simulink model "FusionMODEL_version1"  (R2018a)
settings: Solver=FixedStepAuto  StartTime=0.0  StopTime=SimulationTime  FixedStep=SamplingTime  RelTol=1e-3
undefined symbols (not defined in the file or in its folder): ACTIVATE_CAM, ACTIVATE_RAD, CAM1_detTimeStamp, CAM1_MeasNoise, CAM1_objClassID, CAM1_PX, CAM1_PY, CAM1_VX, CAM1_VY, CAM2_detTimeStamp, CAM2_MeasNoise, CAM2_objClassID, CAM2_PX, CAM2_PY, CAM2_VX, CAM2_VY, CAM3_detTimeStamp, CAM3_MeasNoise, CAM3_objClassID, CAM3_PX, CAM3_PY, CAM3_VX, CAM3_VY, CAM4_detTimeStamp, CAM4_MeasNoise, CAM4_objClassID, CAM4_PX, CAM4_PY, CAM4_VX, CAM4_VY, CAM5_detTimeStamp, CAM5_MeasNoise, CAM5_objClassID, CAM5_PX, CAM5_PY, CAM5_VX, CAM5_VY, CAM6_detTimeStamp, CAM6_MeasNoise, CAM6_objClassID, CAM6_PX, CAM6_PY, CAM6_VX, CAM6_VY, CAM7_detTimeStamp, CAM7_MeasNoise, CAM7_objClassID, CAM7_PX, CAM7_PY, CAM7_VX, CAM7_VY, CAM8_detTimeStamp, CAM8_MeasNoise, CAM8_objClassID, CAM8_PX, CAM8_PY, CAM8_VX, CAM8_VY, CAM_nMeas, CAM_TYPE ... (+151)
libraries: simulink_extras x2
(part 2 of 6)

== system FusionMODEL_version1/OBJECT_TRACKER_SENSOR_FUSION/SPATIAL_ALLIGNMENT/RADAR_MEASUREMENTS_SPATIAL_ALLIGNMENT/SET_MEASUREMENTS ==
  CTSmeasMAT : Inport
  CTSCovMAT : Inport  Port=2
  CTSRefMAT : Inport  Port=3
  validMeasCount : Inport  Port=4
  Add{,1..4} (5 alike) : Sum
  Assignment1 : Assignment  NumberOfDimensions=2  DiagnosticForDimensions=Warning  IndexOptions=Assign all,Starting index (dialog)  Indices=1,1  OutputSizes=1,1
  Assignment2 : Assignment  NumberOfDimensions=3  DiagnosticForDimensions=Warning  IndexOptions=Assign all,Assign all,Starting index (dialog)  Indices=1,1,1  OutputSizes=1,1,1
  Assignment3 : Assignment  NumberOfDimensions=2  DiagnosticForDimensions=Warning  IndexOptions=Assign all,Starting index (dialog)  Indices=1,1  OutputSizes=1,1
  Bus Creator1 : BusCreator  Inputs=5  OutDataTypeStr=Bus: RAD_MEAS_MAT_CTS  NonVirtualBus=on
  Find Nonzero Elements1 : Find  NumberOfInputDimensions=3
  FindNonZeroIndex : MATLAB Function  Commented=on  TreatAsAtomicUnit=on
  Mux1 : Mux  Inputs=6
  Reshape1 : Reshape  OutputDimensionality=Row vector (2-D)
  Selector : Selector  NumberOfDimensions=2  InputPortWidth=3  IndexOptions=Select all,Index vector (dialog)  Indices=1,1  OutputSizes=1,1
  Selector11 : Selector  NumberOfDimensions=2  InputPortWidth=3  IndexOptions=Index vector (dialog),Select all  Indices=1,1  OutputSizes=1,1
  Selector12 : Selector  NumberOfDimensions=2  InputPortWidth=3  IndexOptions=Select all,Index vector (port)  Indices=1,1  OutputSizes=1,1
  Selector14 : Selector  NumberOfDimensions=2  InputPortWidth=3  IndexOptions=Select all,Index vector (port)  Indices=1,1  OutputSizes=1,1
  Selector15 : Selector  NumberOfDimensions=3  InputPortWidth=3  IndexOptions=Select all,Select all,Index vector (port)  Indices=1,1,1  OutputSizes=1,1,1
  Selector2 : Selector  NumberOfDimensions=2  InputPortWidth=3  IndexOptions=Select all,Index vector (dialog)  Indices=5,2  OutputSizes=1,1
  Selector3 : Selector  NumberOfDimensions=2  InputPortWidth=3  IndexOptions=Select all,Index vector (dialog)  Indices=5,3  OutputSizes=1,1
  Selector4 : Selector  NumberOfDimensions=2  InputPortWidth=3  IndexOptions=Select all,Index vector (dialog)  Indices=5,5  OutputSizes=1,1
  Selector5 : Selector  NumberOfDimensions=2  InputPortWidth=3  IndexOptions=Select all,Index vector (dialog)  Indices=6,6  OutputSizes=1,1
  Selector8 : Selector  NumberOfDimensions=2  InputPortWidth=3  IndexOptions=Select all,Index vector (dialog)  Indices=5,4  OutputSizes=1,1
  CTSmeasMATout : Outport
  wires:
  validMeasCount/1 -> Selector2/1, Selector/1, Bus Creator1/4, Selector3/1, Selector8/1, Selector4/1, Selector5/1  "ValidMeasCountMeasCount"
  Add3/1 -> Add4/1, Mux1/5
  Selector3/1 -> Add1/2
  Add2/1 -> Add3/1, Mux1/4
  Add1/1 -> Mux1/3, Add2/1
  Selector4/1 -> Add3/2
  Selector/1 -> Mux1/1, Add/1
  Add/1 -> Add1/1, Mux1/2
  Add4/1 -> Mux1/6
  Selector2/1 -> Add/2
  Selector8/1 -> Add2/2
  Mux1/1 -> Reshape1/1
  Selector5/1 -> Add4/2
  Bus Creator1/1 -> CTSmeasMATout/1
  CTSRefMAT/1 -> [Ref], Selector11/1
  Selector11/1 -> Find Nonzero Elements1/1
  Find Nonzero Elements1/1 -> Selector14/2, Selector12/2, Selector15/2
  CTSmeasMAT/1 -> Assignment1/1, Selector14/1
  Selector14/1 -> Assignment1/2
  Selector15/1 -> Assignment2/2
  Selector12/1 -> Assignment3/2
  CTSCovMAT/1 -> Assignment2/1, Selector15/1
  Assignment3/1 -> Bus Creator1/3  "MeasRef"
  Assignment2/1 -> Bus Creator1/2  "MeasCovariance"
  Assignment1/1 -> Bus Creator1/1  "MeasArray"
  [Ref] -> Assignment3/1, Selector12/1
  Reshape1/1 -> Bus Creator1/5  "ValidCumulativeMeasCount"

== system FusionMODEL_version1/OBJECT_TRACKER_SENSOR_FUSION/SPATIAL_ALLIGNMENT/RADAR_MEASUREMENTS_SPATIAL_ALLIGNMENT/StartingIndexes1 ==
  SnsrCallib : Inport
  CallibrationInfoExtractor : Subsystem
  Subsystem : Subsystem
  StartingIndexes : Outport
  wires:
  CallibrationInfoExtractor/1(R1nMeas) -> Subsystem/1(R1nMeas)
  CallibrationInfoExtractor/2(R2nMeas) -> Subsystem/2(R2nMeas)
  CallibrationInfoExtractor/3(R3nMeas) -> Subsystem/3(R3nMeas)
  CallibrationInfoExtractor/4(R4nMeas) -> Subsystem/4(R4nMeas)
  CallibrationInfoExtractor/5(R5nMeas) -> Subsystem/5(R5nMeas)
  Subsystem/1(StartingIndexes) -> StartingIndexes/1
  SnsrCallib/1 -> CallibrationInfoExtractor/1(SnsrCallib)

== system FusionMODEL_version1/SENSOR_MEASUREMENTS/RADAR_CAMERA_EGO_SENSOR_INTERFACE/CameraSensors/Camera1 ==
  timeIdx : Inport
  nObjCamera : Inport  Port=2
  SensorMeas : Inport  Port=3
  CHECK_IF_DATA_IS_VALID : Subsystem
  GET_DATA : Subsystem
  LOOP_OVER_CAMERAS : ForIterator  ResetStates=reset  IterationSource=external  IterationVariableDataType=int16
  SET_DATA : Subsystem
  Selector : Selector  InputPortWidth=nCameras  IndexOptions=Index vector (dialog)  Indices=1  OutputSizes=1
  C1 : Outport
  wires:
  nObjCamera/1 -> Selector/1
  LOOP_OVER_CAMERAS/1 -> [index]
  GET_DATA/5(OBJ_TYPE) -> SET_DATA/7(OBJ_TYPE)
  [px] -> SET_DATA/2(px)  "px"
  GET_DATA/7(measCaptureTime) -> SET_DATA/9(TIME_STAMP)
  SET_DATA/1(C1) -> C1/1
  [vx] -> SET_DATA/4(vx)  "vx"
  GET_DATA/1(PX) -> CHECK_IF_DATA_IS_VALID/2(px), [px]
  Selector/1 -> LOOP_OVER_CAMERAS/1
  GET_DATA/3(VX) -> CHECK_IF_DATA_IS_VALID/4(vx), [vx]
  timeIdx/1 -> GET_DATA/2(time)
  CHECK_IF_DATA_IS_VALID/1(ID) -> SET_DATA/6(id)
  SensorMeas/1 -> SET_DATA/1(SensorData)
  GET_DATA/6(NOISE_COV) -> SET_DATA/8(NOISE_COV)
  [vy] -> SET_DATA/5(vy)  "vy"
  [py] -> SET_DATA/3(py)  "py"
  GET_DATA/4(VY) -> CHECK_IF_DATA_IS_VALID/5(vy), [vy]
  GET_DATA/2(PY) -> CHECK_IF_DATA_IS_VALID/3(py), [py]
  [index] -> SET_DATA/10(iter), CHECK_IF_DATA_IS_VALID/1(idx), GET_DATA/1(idx)

== system FusionMODEL_version1/SENSOR_MEASUREMENTS/RADAR_CAMERA_EGO_SENSOR_INTERFACE/CameraSensors/Camera2 ==
  timeIdx : Inport
  nObjCamera : Inport  Port=2
  SensorMeas : Inport  Port=3
  ExtractMeasParam1 : Subsystem
  For Iterator : ForIterator  ResetStates=reset  IterationSource=external  IterationVariableDataType=int16
  IsValid2 : Subsystem
  Selector : Selector  InputPortWidth=nCameras  IndexOptions=Starting index (dialog)  Indices=2  OutputSizes=1
  Subsystem1 : Subsystem
  C2 : Outport
  wires:
  ExtractMeasParam1/1(PX) -> IsValid2/2(px), [px]
  ExtractMeasParam1/7(measCaptureTime) -> Subsystem1/9(TIME_STAMP)
  IsValid2/1(ID) -> Subsystem1/6(id)
  [vy] -> Subsystem1/5(vy)  "vy"
  ExtractMeasParam1/6(NOISE_COV) -> Subsystem1/8(NOISE_COV)
  [vx] -> Subsystem1/4(vx)  "vx"
  SensorMeas/1 -> Subsystem1/1(SensorData)
  nObjCamera/1 -> Selector/1
  [py] -> Subsystem1/3(py)  "py"
  For Iterator/1 -> [index]
  [index] -> Subsystem1/10(iter), IsValid2/1(idx), ExtractMeasParam1/1(idx)
  ExtractMeasParam1/4(VY) -> IsValid2/5(vy), [vy]
  [px] -> Subsystem1/2(px)  "px"
  Selector/1 -> For Iterator/1
  ExtractMeasParam1/2(PY) -> IsValid2/3(py), [py]
  Subsystem1/1(C2) -> C2/1
  ExtractMeasParam1/5(OBJ_TYPE) -> Subsystem1/7(OBJ_TYPE)
  timeIdx/1 -> ExtractMeasParam1/2(time)
  ExtractMeasParam1/3(VX) -> IsValid2/4(vx), [vx]

== system FusionMODEL_version1/SENSOR_MEASUREMENTS/RADAR_CAMERA_EGO_SENSOR_INTERFACE/CameraSensors/Camera3 ==
  timeIdx : Inport
  nObjCamera : Inport  Port=2
  SensorMeas : Inport  Port=3
  ExtractMeasParam1 : Subsystem
  For Iterator : ForIterator  ResetStates=reset  IterationSource=external  IterationVariableDataType=int16
  IsValid2 : Subsystem
  Selector : Selector  InputPortWidth=nCameras  IndexOptions=Starting index (dialog)  Indices=3  OutputSizes=1
  Subsystem1 : Subsystem
  C3 : Outport
  wires:
  ExtractMeasParam1/1(PX) -> IsValid2/2(px), [px]
  ExtractMeasParam1/7(measCaptureTime) -> Subsystem1/9(TIME_STAMP)
  IsValid2/1(ID) -> Subsystem1/6(id)
  [vy] -> Subsystem1/5(vy)  "vy"
  ExtractMeasParam1/6(NOISE_COV) -> Subsystem1/8(NOISE_COV)
  [vx] -> Subsystem1/4(vx)  "vx"
  SensorMeas/1 -> Subsystem1/1(SensorData)
  nObjCamera/1 -> Selector/1
  [py] -> Subsystem1/3(py)  "py"
  For Iterator/1 -> [index]
  [index] -> Subsystem1/10(iter), IsValid2/1(idx), ExtractMeasParam1/1(idx)
  ExtractMeasParam1/4(VY) -> IsValid2/5(vy), [vy]
  [px] -> Subsystem1/2(px)  "px"
  Selector/1 -> For Iterator/1
  ExtractMeasParam1/2(PY) -> IsValid2/3(py), [py]
  Subsystem1/1(C3) -> C3/1
  ExtractMeasParam1/5(OBJ_TYPE) -> Subsystem1/7(OBJ_TYPE)
  timeIdx/1 -> ExtractMeasParam1/2(time)
  ExtractMeasParam1/3(VX) -> IsValid2/4(vx), [vx]

== system FusionMODEL_version1/SENSOR_MEASUREMENTS/RADAR_CAMERA_EGO_SENSOR_INTERFACE/CameraSensors/Camera4 ==
  timeIdx : Inport
  nObjCamera : Inport  Port=2
  SensorMeas : Inport  Port=3
  ExtractMeasParam1 : Subsystem
  For Iterator : ForIterator  ResetStates=reset  IterationSource=external  IterationVariableDataType=int16
  IsValid2 : Subsystem
  Selector : Selector  InputPortWidth=nCameras  IndexOptions=Starting index (dialog)  Indices=4  OutputSizes=1
  Subsystem1 : Subsystem
  C4 : Outport
  wires:
  ExtractMeasParam1/1(PX) -> IsValid2/2(px), [px]
  ExtractMeasParam1/7(measCaptureTime) -> Subsystem1/9(TIME_STAMP)
  IsValid2/1(ID) -> Subsystem1/6(id)
  [vy] -> Subsystem1/5(vy)  "vy"
  ExtractMeasParam1/6(NOISE_COV) -> Subsystem1/8(NOISE_COV)
  [vx] -> Subsystem1/4(vx)  "vx"
  SensorMeas/1 -> Subsystem1/1(SensorData)
  nObjCamera/1 -> Selector/1
  [py] -> Subsystem1/3(py)  "py"
  For Iterator/1 -> [index]
  [index] -> Subsystem1/10(iter), IsValid2/1(idx), ExtractMeasParam1/1(idx)
  ExtractMeasParam1/4(VY) -> IsValid2/5(vy), [vy]
  [px] -> Subsystem1/2(px)  "px"
  Selector/1 -> For Iterator/1
  ExtractMeasParam1/2(PY) -> IsValid2/3(py), [py]
  Subsystem1/1(C4) -> C4/1
  ExtractMeasParam1/5(OBJ_TYPE) -> Subsystem1/7(OBJ_TYPE)
  timeIdx/1 -> ExtractMeasParam1/2(time)
  ExtractMeasParam1/3(VX) -> IsValid2/4(vx), [vx]

== system FusionMODEL_version1/SENSOR_MEASUREMENTS/RADAR_CAMERA_EGO_SENSOR_INTERFACE/CameraSensors/Camera5 ==
  timeIdx : Inport
  nObjCamera : Inport  Port=2
  SensorMeas : Inport  Port=3
  ExtractMeasParam1 : Subsystem
  For Iterator : ForIterator  ResetStates=reset  IterationSource=external  IterationVariableDataType=int16
  IsValid2 : Subsystem
  Selector : Selector  InputPortWidth=nCameras  IndexOptions=Starting index (dialog)  Indices=5  OutputSizes=1
  Subsystem1 : Subsystem
  C5 : Outport
  wires:
  ExtractMeasParam1/1(PX) -> IsValid2/2(px), [px]
  ExtractMeasParam1/7(measCaptureTime) -> Subsystem1/9(TIME_STAMP)
  IsValid2/1(ID) -> Subsystem1/6(id)
  [vy] -> Subsystem1/5(vy)  "vy"
  ExtractMeasParam1/6(NOISE_COV) -> Subsystem1/8(NOISE_COV)
  [vx] -> Subsystem1/4(vx)  "vx"
  SensorMeas/1 -> Subsystem1/1(SensorData)
  nObjCamera/1 -> Selector/1
  [py] -> Subsystem1/3(py)  "py"
  For Iterator/1 -> [index]
  [index] -> Subsystem1/10(iter), IsValid2/1(idx), ExtractMeasParam1/1(idx)
  ExtractMeasParam1/4(VY) -> IsValid2/5(vy), [vy]
  [px] -> Subsystem1/2(px)  "px"
  Selector/1 -> For Iterator/1
  ExtractMeasParam1/2(PY) -> IsValid2/3(py), [py]
  Subsystem1/1(C5) -> C5/1
  ExtractMeasParam1/5(OBJ_TYPE) -> Subsystem1/7(OBJ_TYPE)
  timeIdx/1 -> ExtractMeasParam1/2(time)
  ExtractMeasParam1/3(VX) -> IsValid2/4(vx), [vx]

== system FusionMODEL_version1/SENSOR_MEASUREMENTS/RADAR_CAMERA_EGO_SENSOR_INTERFACE/CameraSensors/Camera6 ==
  timeIdx : Inport
  nObjCamera : Inport  Port=2
  SensorMeas : Inport  Port=3
  ExtractMeasParam1 : Subsystem
  For Iterator : ForIterator  ResetStates=reset  IterationSource=external  IterationVariableDataType=int16
  IsValid2 : Subsystem
  Selector : Selector  InputPortWidth=nCameras  IndexOptions=Starting index (dialog)  Indices=6  OutputSizes=1
  Subsystem1 : Subsystem
  C6 : Outport
  wires:
  ExtractMeasParam1/1(PX) -> IsValid2/2(px), [px]
  ExtractMeasParam1/7(measCaptureTime) -> Subsystem1/9(TIME_STAMP)
  IsValid2/1(ID) -> Subsystem1/6(id)
  [vy] -> Subsystem1/5(vy)  "vy"
  ExtractMeasParam1/6(NOISE_COV) -> Subsystem1/8(NOISE_COV)
  [vx] -> Subsystem1/4(vx)  "vx"
  SensorMeas/1 -> Subsystem1/1(SensorData)
  nObjCamera/1 -> Selector/1
  [py] -> Subsystem1/3(py)  "py"
  For Iterator/1 -> [index]
  [index] -> Subsystem1/10(iter), IsValid2/1(idx), ExtractMeasParam1/1(idx)
  ExtractMeasParam1/4(VY) -> IsValid2/5(vy), [vy]
  [px] -> Subsystem1/2(px)  "px"
  Selector/1 -> For Iterator/1
  ExtractMeasParam1/2(PY) -> IsValid2/3(py), [py]
  Subsystem1/1(C6) -> C6/1
  ExtractMeasParam1/5(OBJ_TYPE) -> Subsystem1/7(OBJ_TYPE)
  timeIdx/1 -> ExtractMeasParam1/2(time)
  ExtractMeasParam1/3(VX) -> IsValid2/4(vx), [vx]

== system FusionMODEL_version1/SENSOR_MEASUREMENTS/RADAR_CAMERA_EGO_SENSOR_INTERFACE/CameraSensors/Camera7 ==
  timeIdx : Inport
  nObjCamera : Inport  Port=2
  SensorMeas : Inport  Port=3
  ExtractMeasParam1 : Subsystem
  For Iterator : ForIterator  ResetStates=reset  IterationSource=external  IterationVariableDataType=int16
  IsValid2 : Subsystem
  Selector : Selector  InputPortWidth=nCameras  IndexOptions=Starting index (dialog)  Indices=7  OutputSizes=1
  Subsystem1 : Subsystem
  C7 : Outport
  wires:
  ExtractMeasParam1/1(PX) -> IsValid2/2(px), [px]
  ExtractMeasParam1/7(measCaptureTime) -> Subsystem1/9(TIME_STAMP)
  IsValid2/1(ID) -> Subsystem1/6(id)
  [vy] -> Subsystem1/5(vy)  "vy"
  ExtractMeasParam1/6(NOISE_COV) -> Subsystem1/8(NOISE_COV)
  [vx] -> Subsystem1/4(vx)  "vx"
  SensorMeas/1 -> Subsystem1/1(SensorData)
  nObjCamera/1 -> Selector/1
  [py] -> Subsystem1/3(py)  "py"
  For Iterator/1 -> [index]
  [index] -> Subsystem1/10(iter), IsValid2/1(idx), ExtractMeasParam1/1(idx)
  ExtractMeasParam1/4(VY) -> IsValid2/5(vy), [vy]
  [px] -> Subsystem1/2(px)  "px"
  Selector/1 -> For Iterator/1
  ExtractMeasParam1/2(PY) -> IsValid2/3(py), [py]
  Subsystem1/1(C7) -> C7/1
  ExtractMeasParam1/5(OBJ_TYPE) -> Subsystem1/7(OBJ_TYPE)
  timeIdx/1 -> ExtractMeasParam1/2(time)
  ExtractMeasParam1/3(VX) -> IsValid2/4(vx), [vx]

== system FusionMODEL_version1/SENSOR_MEASUREMENTS/RADAR_CAMERA_EGO_SENSOR_INTERFACE/CameraSensors/Camera8 ==
  timeIdx : Inport
  nObjCamera : Inport  Port=2
  SensorMeas : Inport  Port=3
  ExtractMeasParam1 : Subsystem
  For Iterator : ForIterator  ResetStates=reset  IterationSource=external  IterationVariableDataType=int16
  IsValid2 : Subsystem
  Selector : Selector  InputPortWidth=nCameras  IndexOptions=Starting index (dialog)  Indices=8  OutputSizes=1
  Subsystem1 : Subsystem
  C8 : Outport
  wires:
  ExtractMeasParam1/1(PX) -> IsValid2/2(px), [px]
  ExtractMeasParam1/7(measCaptureTime) -> Subsystem1/9(TIME_STAMP)
  IsValid2/1(ID) -> Subsystem1/6(id)
  [vy] -> Subsystem1/5(vy)  "vy"
  ExtractMeasParam1/6(NOISE_COV) -> Subsystem1/8(NOISE_COV)
  [vx] -> Subsystem1/4(vx)  "vx"
  SensorMeas/1 -> Subsystem1/1(SensorData)
  nObjCamera/1 -> Selector/1
  [py] -> Subsystem1/3(py)  "py"
  For Iterator/1 -> [index]
  [index] -> Subsystem1/10(iter), IsValid2/1(idx), ExtractMeasParam1/1(idx)
  ExtractMeasParam1/4(VY) -> IsValid2/5(vy), [vy]
  [px] -> Subsystem1/2(px)  "px"
  Selector/1 -> For Iterator/1
  ExtractMeasParam1/2(PY) -> IsValid2/3(py), [py]
  Subsystem1/1(C8) -> C8/1
  ExtractMeasParam1/5(OBJ_TYPE) -> Subsystem1/7(OBJ_TYPE)
  timeIdx/1 -> ExtractMeasParam1/2(time)
  ExtractMeasParam1/3(VX) -> IsValid2/4(vx), [vx]

== system FusionMODEL_version1/SENSOR_MEASUREMENTS/RADAR_CAMERA_EGO_SENSOR_INTERFACE/EgoSensors/ExtractMeasParam ==
  timeIdx : Inport
  Constant : Constant  Value=EGO_PX
  Constant1 : Constant  Value=EGO_PY
  Constant2 : Constant  Value=EGO_VX
  Constant3 : Constant  Value=EGO_VY
  Constant4 : Constant  Value=EGO_YAW
  Constant5 : Constant  Value=EGO_YAWRATE
  Constant6 : Constant  Value=EGO_TimeStamp
  Constant7 : Constant  Value=EGO_IgnitionStatus
  EGO_PX : Selector  NumberOfDimensions=2  InputPortWidth=portSize  IndexOptions=Select all,Index vector (port)  Indices=[1 3],1  OutputSizes=1,1
  EGO_PY : Selector  NumberOfDimensions=2  InputPortWidth=portSize  IndexOptions=Select all,Index vector (port)  Indices=[1 3],1  OutputSizes=1,1
  EGO_VX : Selector  NumberOfDimensions=2  InputPortWidth=portSize  IndexOptions=Select all,Index vector (port)  Indices=[1 3],1  OutputSizes=1,1
  EGO_VY : Selector  NumberOfDimensions=2  InputPortWidth=portSize  IndexOptions=Select all,Index vector (port)  Indices=[1 3],1  OutputSizes=1,1
  EGO_YAW : Selector  NumberOfDimensions=2  InputPortWidth=portSize  IndexOptions=Select all,Index vector (port)  Indices=[1 3],1  OutputSizes=1,1
  EGO_YAWRATE : Selector  NumberOfDimensions=2  InputPortWidth=portSize  IndexOptions=Select all,Index vector (port)  Indices=[1 3],1  OutputSizes=1,1
  TIME_STAMP : Selector  NumberOfDimensions=2  InputPortWidth=portSize  IndexOptions=Select all,Index vector (port)  Indices=[1 3],1  OutputSizes=1,1
  TIME_STAMP1 : Selector  NumberOfDimensions=2  InputPortWidth=portSize  IndexOptions=Select all,Index vector (port)  Indices=[1 3],1  OutputSizes=1,1
  EgoTimeStamp : Outport
  EgoPx : Outport  Port=2
  EgoPy : Outport  Port=3
  EgoVx : Outport  Port=4
  EgoVy : Outport  Port=5
  EgoYaw : Outport  Port=6
  EgoYawRate : Outport  Port=7
  EgoIgnitionStatus : Outport  Port=8
  wires:
  Constant3/1 -> EGO_VY/1
  Constant2/1 -> EGO_VX/1
  Constant/1 -> EGO_PX/1
  Constant1/1 -> EGO_PY/1
  EGO_VX/1 -> EgoVx/1
  EGO_PX/1 -> EgoPx/1
  timeIdx/1 -> EGO_PX/2, EGO_PY/2, EGO_VX/2, EGO_VY/2, EGO_YAW/2, EGO_YAWRATE/2, TIME_STAMP1/2, TIME_STAMP/2
  Constant4/1 -> EGO_YAW/1
  EGO_YAW/1 -> EgoYaw/1
  Constant6/1 -> TIME_STAMP/1
  TIME_STAMP/1 -> EgoTimeStamp/1
  EGO_YAWRATE/1 -> EgoYawRate/1
  Constant5/1 -> EGO_YAWRATE/1
  EGO_PY/1 -> EgoPy/1
  EGO_VY/1 -> EgoVy/1
  Constant7/1 -> TIME_STAMP1/1
  TIME_STAMP1/1 -> EgoIgnitionStatus/1

== system FusionMODEL_version1/SENSOR_MEASUREMENTS/RADAR_CAMERA_EGO_SENSOR_INTERFACE/RadarSensors/Radar1 ==
  timeIdx : Inport
  nObjRadar : Inport  Port=2
  SensorMeas : Inport  Port=3
  CHECK_IF_DATA_VALID : Subsystem
  GET_DATA : Subsystem
  LOOP_OVER_RADARS : ForIterator  ResetStates=reset  IterationSource=external  IterationVariableDataType=int16
  SET_DATA : Subsystem
  Selector : Selector  InputPortWidth=nRadars  IndexOptions=Starting index (dialog)  Indices=1  OutputSizes=1
  R1 : Outport
  wires:
  nObjRadar/1 -> Selector/1
  LOOP_OVER_RADARS/1 -> [index]
  [index] -> CHECK_IF_DATA_VALID/1(idx), GET_DATA/1(idx), SET_DATA/10(iter)
  timeIdx/1 -> GET_DATA/2(time)
  GET_DATA/1(PX) -> CHECK_IF_DATA_VALID/2(px), [px]
  GET_DATA/2(PY) -> CHECK_IF_DATA_VALID/3(py), [py]
  GET_DATA/3(VX) -> CHECK_IF_DATA_VALID/4(vx), [vx]
  GET_DATA/4(VY) -> CHECK_IF_DATA_VALID/5(vy), [vy]
  SensorMeas/1 -> SET_DATA/1(SensorData)
  [px] -> SET_DATA/2(px)  "px"
  [py] -> SET_DATA/3(py)  "py"
  [vx] -> SET_DATA/4(vx)  "vx"
  [vy] -> SET_DATA/5(vy)  "vy"
  SET_DATA/1(R1) -> R1/1
  CHECK_IF_DATA_VALID/1(ID) -> SET_DATA/6(id)
  Selector/1 -> LOOP_OVER_RADARS/1
  GET_DATA/5(SNR) -> SET_DATA/7(SNR)
  GET_DATA/6(NOISE_COV) -> SET_DATA/8(NOISE_COV)
  GET_DATA/7(measCaptureTime) -> SET_DATA/9(TIME_STAMP)

== system FusionMODEL_version1/SENSOR_MEASUREMENTS/RADAR_CAMERA_EGO_SENSOR_INTERFACE/RadarSensors/Radar2 ==
  timeIdx : Inport
  nObjRadar : Inport  Port=2
  SensorMeas : Inport  Port=3
  ExtractMeasParam : Subsystem
  For Iterator : ForIterator  ResetStates=reset  IterationSource=external  IterationVariableDataType=int16
  IsValid1 : Subsystem
  Selector : Selector  InputPortWidth=nRadars  IndexOptions=Starting index (dialog)  Indices=2  OutputSizes=1
  Subsystem : Subsystem
  R2 : Outport
  wires:
  [vx] -> Subsystem/4(vx)  "vx"
  Subsystem/1(R2) -> R2/1
  ExtractMeasParam/1(PX) -> IsValid1/2(px), [px]
  IsValid1/1(ID) -> Subsystem/6(id)
  [py] -> Subsystem/3(py)  "py"
  ExtractMeasParam/3(VX) -> IsValid1/4(vx), [vx]
  ExtractMeasParam/6(NOISE_COV) -> Subsystem/8(NOISE_COV)
  ExtractMeasParam/4(VY) -> IsValid1/5(vy), [vy]
  [px] -> Subsystem/2(px)  "px"
  nObjRadar/1 -> Selector/1
  SensorMeas/1 -> Subsystem/1(SensorData)
  timeIdx/1 -> ExtractMeasParam/2(time)
  [index] -> IsValid1/1(idx), ExtractMeasParam/1(idx), Subsystem/10(iter)
  [vy] -> Subsystem/5(vy)  "vy"
  ExtractMeasParam/2(PY) -> IsValid1/3(py), [py]
  For Iterator/1 -> [index]
  ExtractMeasParam/5(SNR) -> Subsystem/7(SNR)
  ExtractMeasParam/7(measCaptureTime) -> Subsystem/9(TIME_STAMP)
  Selector/1 -> For Iterator/1

== system FusionMODEL_version1/SENSOR_MEASUREMENTS/RADAR_CAMERA_EGO_SENSOR_INTERFACE/RadarSensors/Radar3 ==
  timeIdx : Inport
  nObjRadar : Inport  Port=2
  SensorMeas : Inport  Port=3
  ExtractMeasParam : Subsystem
  For Iterator : ForIterator  ResetStates=reset  IterationSource=external  IterationVariableDataType=int16
  IsValid1 : Subsystem
  Selector : Selector  InputPortWidth=nRadars  IndexOptions=Starting index (dialog)  Indices=3  OutputSizes=1
  Subsystem : Subsystem
  R3 : Outport
  wires:
  [vx] -> Subsystem/4(vx)  "vx"
  Subsystem/1(R3) -> R3/1
  ExtractMeasParam/1(PX) -> IsValid1/2(px), [px]
  IsValid1/1(ID) -> Subsystem/6(id)
  [py] -> Subsystem/3(py)  "py"
  ExtractMeasParam/3(VX) -> IsValid1/4(vx), [vx]
  ExtractMeasParam/6(NOISE_COV) -> Subsystem/8(NOISE_COV)
  ExtractMeasParam/4(VY) -> IsValid1/5(vy), [vy]
  [px] -> Subsystem/2(px)  "px"
  nObjRadar/1 -> Selector/1
  SensorMeas/1 -> Subsystem/1(SensorData)
  timeIdx/1 -> ExtractMeasParam/2(time)
  [index] -> IsValid1/1(idx), ExtractMeasParam/1(idx), Subsystem/10(iter)
  [vy] -> Subsystem/5(vy)  "vy"
  ExtractMeasParam/2(PY) -> IsValid1/3(py), [py]
  For Iterator/1 -> [index]
  ExtractMeasParam/5(SNR) -> Subsystem/7(SNR)
  ExtractMeasParam/7(measCaptureTime) -> Subsystem/9(TIME_STAMP)
  Selector/1 -> For Iterator/1

== system FusionMODEL_version1/SENSOR_MEASUREMENTS/RADAR_CAMERA_EGO_SENSOR_INTERFACE/RadarSensors/Radar4 ==
  timeIdx : Inport
  nObjRadar : Inport  Port=2
  SensorMeas : Inport  Port=3
  ExtractMeasParam : Subsystem
  For Iterator : ForIterator  ResetStates=reset  IterationSource=external  IterationVariableDataType=int16
  IsValid1 : Subsystem
  Selector : Selector  InputPortWidth=nRadars  IndexOptions=Starting index (dialog)  Indices=4  OutputSizes=1
  Subsystem : Subsystem
  R4 : Outport
  wires:
  ExtractMeasParam/2(PY) -> IsValid1/3(py), [py]
  [vy] -> Subsystem/5(vy)  "vy"
  [index] -> IsValid1/1(idx), ExtractMeasParam/1(idx), Subsystem/10(iter)
  SensorMeas/1 -> Subsystem/1(SensorData)
  ExtractMeasParam/6(NOISE_COV) -> Subsystem/8(NOISE_COV)
  ExtractMeasParam/4(VY) -> IsValid1/5(vy), [vy]
  ExtractMeasParam/3(VX) -> IsValid1/4(vx), [vx]
  timeIdx/1 -> ExtractMeasParam/2(time)
  IsValid1/1(ID) -> Subsystem/6(id)
  ExtractMeasParam/1(PX) -> IsValid1/2(px), [px]
  [vx] -> Subsystem/4(vx)  "vx"
  Selector/1 -> For Iterator/1
  nObjRadar/1 -> Selector/1
  Subsystem/1(R4) -> R4/1
  ExtractMeasParam/7(measCaptureTime) -> Subsystem/9(TIME_STAMP)
  [px] -> Subsystem/2(px)  "px"
  ExtractMeasParam/5(SNR) -> Subsystem/7(SNR)
  [py] -> Subsystem/3(py)  "py"
  For Iterator/1 -> [index]

== system FusionMODEL_version1/SENSOR_MEASUREMENTS/RADAR_CAMERA_EGO_SENSOR_INTERFACE/RadarSensors/Radar5 ==
  timeIdx : Inport
  nObjRadar : Inport  Port=2
  SensorMeas : Inport  Port=3
  ExtractMeasParam : Subsystem
  For Iterator : ForIterator  ResetStates=reset  IterationSource=external  IterationVariableDataType=int16
  IsValid1 : Subsystem
  Selector : Selector  InputPortWidth=nRadars  IndexOptions=Starting index (dialog)  Indices=5  OutputSizes=1
  Subsystem : Subsystem
  R5 : Outport
  wires:
  ExtractMeasParam/2(PY) -> IsValid1/3(py), [py]
  [vy] -> Subsystem/5(vy)  "vy"
  [index] -> IsValid1/1(idx), ExtractMeasParam/1(idx), Subsystem/10(iter)
  SensorMeas/1 -> Subsystem/1(SensorData)
  ExtractMeasParam/6(NOISE_COV) -> Subsystem/8(NOISE_COV)
  ExtractMeasParam/4(VY) -> IsValid1/5(vy), [vy]
  ExtractMeasParam/3(VX) -> IsValid1/4(vx), [vx]
  timeIdx/1 -> ExtractMeasParam/2(time)
  IsValid1/1(ID) -> Subsystem/6(id)
  ExtractMeasParam/1(PX) -> IsValid1/2(px), [px]
  [vx] -> Subsystem/4(vx)  "vx"
  Selector/1 -> For Iterator/1
  nObjRadar/1 -> Selector/1
  Subsystem/1(R5) -> R5/1
  ExtractMeasParam/7(measCaptureTime) -> Subsystem/9(TIME_STAMP)
  [px] -> Subsystem/2(px)  "px"
  ExtractMeasParam/5(SNR) -> Subsystem/7(SNR)
  [py] -> Subsystem/3(py)  "py"
  For Iterator/1 -> [index]

== system FusionMODEL_version1/SENSOR_MEASUREMENTS/RADAR_CAMERA_EGO_SENSOR_INTERFACE/RadarSensors/Radar6 ==
  timeIdx : Inport
  nObjRadar : Inport  Port=2
  SensorMeas : Inport  Port=3
  ExtractMeasParam : Subsystem
  For Iterator : ForIterator  ResetStates=reset  IterationSource=external  IterationVariableDataType=int16
  IsValid1 : Subsystem
  Selector : Selector  InputPortWidth=nRadars  IndexOptions=Starting index (dialog)  Indices=6  OutputSizes=1
  Subsystem : Subsystem
  R6 : Outport
  wires:
  ExtractMeasParam/2(PY) -> IsValid1/3(py), [py]
  [vy] -> Subsystem/5(vy)  "vy"
  [index] -> IsValid1/1(idx), ExtractMeasParam/1(idx), Subsystem/10(iter)
  SensorMeas/1 -> Subsystem/1(SensorData)
  ExtractMeasParam/6(NOISE_COV) -> Subsystem/8(NOISE_COV)
  ExtractMeasParam/4(VY) -> IsValid1/5(vy), [vy]
  ExtractMeasParam/3(VX) -> IsValid1/4(vx), [vx]
  timeIdx/1 -> ExtractMeasParam/2(time)
  IsValid1/1(ID) -> Subsystem/6(id)
  ExtractMeasParam/1(PX) -> IsValid1/2(px), [px]
  [vx] -> Subsystem/4(vx)  "vx"
  Selector/1 -> For Iterator/1
  nObjRadar/1 -> Selector/1
  Subsystem/1(R6) -> R6/1
  ExtractMeasParam/7(measCaptureTime) -> Subsystem/9(TIME_STAMP)
  [px] -> Subsystem/2(px)  "px"
  ExtractMeasParam/5(SNR) -> Subsystem/7(SNR)
  [py] -> Subsystem/3(py)  "py"
  For Iterator/1 -> [index]

== system FusionMODEL_version1/SENSOR_MEASUREMENTS/RADAR_CAMERA_EGO_SENSOR_INTERFACE/RoadSensors/Camera1 ==
  timeIdx : Inport
  nLines : Inport  Port=2
  CameraLineCoeff : Inport  Port=3
  CHECK_IF_DATA_IS_VALID : Subsystem
  GET_DATA : Subsystem
  LOOP_OVER_CAMERAS : ForIterator  ResetStates=reset  IterationSource=external  IterationVariableDataType=int16
  SET_DATA : Subsystem
  Selector : Selector  InputPortWidth=nCameras  IndexOptions=Index vector (dialog)  Indices=1  OutputSizes=1
  C1 : Outport
  wires:
  nLines/1 -> Selector/1
  LOOP_OVER_CAMERAS/1 -> [index]
  GET_DATA/5(lateralOffset) -> SET_DATA/7(lateralOffset)
  [curv] -> SET_DATA/2(curv)
  GET_DATA/9(measCaptureTime) -> SET_DATA/11(TIME_STAMP)
  SET_DATA/1(C1) -> C1/1
  [curvLen] -> SET_DATA/4(curvLen)
  GET_DATA/1(curvature) -> CHECK_IF_DATA_IS_VALID/2(curvature), [curv]
  Selector/1 -> LOOP_OVER_CAMERAS/1
  GET_DATA/3(curvLength) -> CHECK_IF_DATA_IS_VALID/4(curvLength), [curvLen]
  timeIdx/1 -> GET_DATA/2(time)
  CHECK_IF_DATA_IS_VALID/1(validID) -> SET_DATA/6(ValidID)
  CameraLineCoeff/1 -> SET_DATA/1(CameraLineCoeff)
  GET_DATA/6(xmin) -> SET_DATA/8(xmin)
  [alpha] -> SET_DATA/5(alpha)
  [curvRate] -> SET_DATA/3(curvRate)
  GET_DATA/4(headingAngle) -> CHECK_IF_DATA_IS_VALID/5(HeadingAngle), [alpha]
  GET_DATA/2(curvRate) -> CHECK_IF_DATA_IS_VALID/3(curvatureRate), [curvRate]
  [index] -> CHECK_IF_DATA_IS_VALID/1(LineID), SET_DATA/12(iter), GET_DATA/1(idx)
  GET_DATA/7(xmax) -> SET_DATA/9(xmax)
  GET_DATA/8(lineMarkWidth) -> SET_DATA/10(lineWidth)

== system FusionMODEL_version1/SENSOR_MEASUREMENTS/RADAR_CAMERA_EGO_SENSOR_INTERFACE/RoadSensors/Camera2 ==
  timeIdx : Inport
  nLines : Inport  Port=2
  CameraLineCoeff : Inport  Port=3
  ExtractMeasParam1 : Subsystem
  For Iterator : ForIterator  ResetStates=reset  IterationSource=external  IterationVariableDataType=int16
  IsValid2 : Subsystem
  Selector : Selector  InputPortWidth=nCameras  IndexOptions=Index vector (dialog)  Indices=2  OutputSizes=1
  Subsystem1 : Subsystem
  C1 : Outport
  wires:
  ExtractMeasParam1/7(xmax) -> Subsystem1/9(xmax)
  ExtractMeasParam1/8(lineMarkWidth) -> Subsystem1/10(lineWidth)
  [index] -> IsValid2/1(LineID), Subsystem1/12(iter), ExtractMeasParam1/1(idx)
  timeIdx/1 -> ExtractMeasParam1/2(time)
  ExtractMeasParam1/2(curvRate) -> IsValid2/3(curvatureRate), [curvRate]
  [curvRate] -> Subsystem1/3(curvRate)
  [curv] -> Subsystem1/2(curv)
  ExtractMeasParam1/3(curvLength) -> IsValid2/4(curvLength), [curvLen]
  ExtractMeasParam1/1(curvature) -> IsValid2/2(curvature), [curv]
  Subsystem1/1(C1) -> C1/1
  [curvLen] -> Subsystem1/4(curvLen)
  For Iterator/1 -> [index]
  ExtractMeasParam1/4(headingAngle) -> IsValid2/5(HeadingAngle), [alpha]
  ExtractMeasParam1/5(lateralOffset) -> Subsystem1/7(lateralOffset)
  Selector/1 -> For Iterator/1
  IsValid2/1(validID) -> Subsystem1/6(ValidID)
  ExtractMeasParam1/6(xmin) -> Subsystem1/8(xmin)
  CameraLineCoeff/1 -> Subsystem1/1(CameraLineCoeff)
  nLines/1 -> Selector/1
  ExtractMeasParam1/9(measCaptureTime) -> Subsystem1/11(TIME_STAMP)
  [alpha] -> Subsystem1/5(alpha)

== system FusionMODEL_version1/SENSOR_MEASUREMENTS/RADAR_CAMERA_EGO_SENSOR_INTERFACE/RoadSensors/Camera3 ==
  timeIdx : Inport
  nLines : Inport  Port=2
  CameraLineCoeff : Inport  Port=3
  ExtractMeasParam1 : Subsystem
  For Iterator : ForIterator  ResetStates=reset  IterationSource=external  IterationVariableDataType=int16
  IsValid2 : Subsystem
  Selector : Selector  InputPortWidth=nCameras  IndexOptions=Index vector (dialog)  Indices=3  OutputSizes=1
  Subsystem1 : Subsystem
  C1 : Outport
  wires:
  ExtractMeasParam1/7(xmax) -> Subsystem1/9(xmax)
  ExtractMeasParam1/8(lineMarkWidth) -> Subsystem1/10(lineWidth)
  [index] -> IsValid2/1(LineID), Subsystem1/12(iter), ExtractMeasParam1/1(idx)
  timeIdx/1 -> ExtractMeasParam1/2(time)
  ExtractMeasParam1/2(curvRate) -> IsValid2/3(curvatureRate), [curvRate]
  [curvRate] -> Subsystem1/3(curvRate)
  [curv] -> Subsystem1/2(curv)
  ExtractMeasParam1/3(curvLength) -> IsValid2/4(curvLength), [curvLen]
  ExtractMeasParam1/1(curvature) -> IsValid2/2(curvature), [curv]
  Subsystem1/1(C1) -> C1/1
  [curvLen] -> Subsystem1/4(curvLen)
  For Iterator/1 -> [index]
  ExtractMeasParam1/4(headingAngle) -> IsValid2/5(HeadingAngle), [alpha]
  ExtractMeasParam1/5(lateralOffset) -> Subsystem1/7(lateralOffset)
  Selector/1 -> For Iterator/1
  IsValid2/1(validID) -> Subsystem1/6(ValidID)
  ExtractMeasParam1/6(xmin) -> Subsystem1/8(xmin)
  CameraLineCoeff/1 -> Subsystem1/1(CameraLineCoeff)
  nLines/1 -> Selector/1
  ExtractMeasParam1/9(measCaptureTime) -> Subsystem1/11(TIME_STAMP)
  [alpha] -> Subsystem1/5(alpha)

== system FusionMODEL_version1/SENSOR_MEASUREMENTS/RADAR_CAMERA_EGO_SENSOR_INTERFACE/RoadSensors/Camera4 ==
  timeIdx : Inport
  nLines : Inport  Port=2
  CameraLineCoeff : Inport  Port=3
  ExtractMeasParam1 : Subsystem
  For Iterator : ForIterator  ResetStates=reset  IterationSource=external  IterationVariableDataType=int16
  IsValid2 : Subsystem
  Selector : Selector  InputPortWidth=nCameras  IndexOptions=Index vector (dialog)  Indices=4  OutputSizes=1
  Subsystem1 : Subsystem
  C1 : Outport
  wires:
  ExtractMeasParam1/7(xmax) -> Subsystem1/9(xmax)
  ExtractMeasParam1/8(lineMarkWidth) -> Subsystem1/10(lineWidth)
  [index] -> IsValid2/1(LineID), Subsystem1/12(iter), ExtractMeasParam1/1(idx)
  timeIdx/1 -> ExtractMeasParam1/2(time)
  ExtractMeasParam1/2(curvRate) -> IsValid2/3(curvatureRate), [curvRate]
  [curvRate] -> Subsystem1/3(curvRate)
  [curv] -> Subsystem1/2(curv)
  ExtractMeasParam1/3(curvLength) -> IsValid2/4(curvLength), [curvLen]
  ExtractMeasParam1/1(curvature) -> IsValid2/2(curvature), [curv]
  Subsystem1/1(C1) -> C1/1
  [curvLen] -> Subsystem1/4(curvLen)
  For Iterator/1 -> [index]
  ExtractMeasParam1/4(headingAngle) -> IsValid2/5(HeadingAngle), [alpha]
  ExtractMeasParam1/5(lateralOffset) -> Subsystem1/7(lateralOffset)
  Selector/1 -> For Iterator/1
  IsValid2/1(validID) -> Subsystem1/6(ValidID)
  ExtractMeasParam1/6(xmin) -> Subsystem1/8(xmin)
  CameraLineCoeff/1 -> Subsystem1/1(CameraLineCoeff)
  nLines/1 -> Selector/1
  ExtractMeasParam1/9(measCaptureTime) -> Subsystem1/11(TIME_STAMP)
  [alpha] -> Subsystem1/5(alpha)

== system FusionMODEL_version1/SENSOR_MEASUREMENTS/RADAR_CAMERA_EGO_SENSOR_INTERFACE/RoadSensors/Camera5 ==
  timeIdx : Inport
  nLines : Inport  Port=2
  CameraLineCoeff : Inport  Port=3
  ExtractMeasParam1 : Subsystem
  For Iterator : ForIterator  ResetStates=reset  IterationSource=external  IterationVariableDataType=int16
  IsValid2 : Subsystem
  Selector : Selector  InputPortWidth=nCameras  IndexOptions=Index vector (dialog)  Indices=5  OutputSizes=1
  Subsystem1 : Subsystem
  C1 : Outport
  wires:
  ExtractMeasParam1/7(xmax) -> Subsystem1/9(xmax)
  ExtractMeasParam1/8(lineMarkWidth) -> Subsystem1/10(lineWidth)
  [index] -> IsValid2/1(LineID), Subsystem1/12(iter), ExtractMeasParam1/1(idx)
  timeIdx/1 -> ExtractMeasParam1/2(time)
  ExtractMeasParam1/2(curvRate) -> IsValid2/3(curvatureRate), [curvRate]
  [curvRate] -> Subsystem1/3(curvRate)
  [curv] -> Subsystem1/2(curv)
  ExtractMeasParam1/3(curvLength) -> IsValid2/4(curvLength), [curvLen]
  ExtractMeasParam1/1(curvature) -> IsValid2/2(curvature), [curv]
  Subsystem1/1(C1) -> C1/1
  [curvLen] -> Subsystem1/4(curvLen)
  For Iterator/1 -> [index]
  ExtractMeasParam1/4(headingAngle) -> IsValid2/5(HeadingAngle), [alpha]
  ExtractMeasParam1/5(lateralOffset) -> Subsystem1/7(lateralOffset)
  Selector/1 -> For Iterator/1
  IsValid2/1(validID) -> Subsystem1/6(ValidID)
  ExtractMeasParam1/6(xmin) -> Subsystem1/8(xmin)
  CameraLineCoeff/1 -> Subsystem1/1(CameraLineCoeff)
  nLines/1 -> Selector/1
  ExtractMeasParam1/9(measCaptureTime) -> Subsystem1/11(TIME_STAMP)
  [alpha] -> Subsystem1/5(alpha)

== system FusionMODEL_version1/SENSOR_MEASUREMENTS/RADAR_CAMERA_EGO_SENSOR_INTERFACE/RoadSensors/Camera6 ==
  timeIdx : Inport
  nLines : Inport  Port=2
  CameraLineCoeff : Inport  Port=3
  ExtractMeasParam1 : Subsystem
  For Iterator : ForIterator  ResetStates=reset  IterationSource=external  IterationVariableDataType=int16
  IsValid2 : Subsystem
  Selector : Selector  InputPortWidth=nCameras  IndexOptions=Index vector (dialog)  Indices=6  OutputSizes=1
  Subsystem1 : Subsystem
  C1 : Outport
  wires:
  ExtractMeasParam1/7(xmax) -> Subsystem1/9(xmax)
  ExtractMeasParam1/8(lineMarkWidth) -> Subsystem1/10(lineWidth)
  [index] -> IsValid2/1(LineID), Subsystem1/12(iter), ExtractMeasParam1/1(idx)
  timeIdx/1 -> ExtractMeasParam1/2(time)
  ExtractMeasParam1/2(curvRate) -> IsValid2/3(curvatureRate), [curvRate]
  [curvRate] -> Subsystem1/3(curvRate)
  [curv] -> Subsystem1/2(curv)
  ExtractMeasParam1/3(curvLength) -> IsValid2/4(curvLength), [curvLen]
  ExtractMeasParam1/1(curvature) -> IsValid2/2(curvature), [curv]
  Subsystem1/1(C1) -> C1/1
  [curvLen] -> Subsystem1/4(curvLen)
  For Iterator/1 -> [index]
  ExtractMeasParam1/4(headingAngle) -> IsValid2/5(HeadingAngle), [alpha]
  ExtractMeasParam1/5(lateralOffset) -> Subsystem1/7(lateralOffset)
  Selector/1 -> For Iterator/1
  IsValid2/1(validID) -> Subsystem1/6(ValidID)
  ExtractMeasParam1/6(xmin) -> Subsystem1/8(xmin)
  CameraLineCoeff/1 -> Subsystem1/1(CameraLineCoeff)
  nLines/1 -> Selector/1
  ExtractMeasParam1/9(measCaptureTime) -> Subsystem1/11(TIME_STAMP)
  [alpha] -> Subsystem1/5(alpha)

== system FusionMODEL_version1/SENSOR_MEASUREMENTS/RADAR_CAMERA_EGO_SENSOR_INTERFACE/RoadSensors/Camera7 ==
  timeIdx : Inport
  nLines : Inport  Port=2
  CameraLineCoeff : Inport  Port=3
  ExtractMeasParam1 : Subsystem
  For Iterator : ForIterator  ResetStates=reset  IterationSource=external  IterationVariableDataType=int16
  IsValid2 : Subsystem
  Selector : Selector  InputPortWidth=nCameras  IndexOptions=Index vector (dialog)  Indices=7  OutputSizes=1
  Subsystem1 : Subsystem
  C1 : Outport
  wires:
  ExtractMeasParam1/7(xmax) -> Subsystem1/9(xmax)
  ExtractMeasParam1/8(lineMarkWidth) -> Subsystem1/10(lineWidth)
  [index] -> IsValid2/1(LineID), Subsystem1/12(iter), ExtractMeasParam1/1(idx)
  timeIdx/1 -> ExtractMeasParam1/2(time)
  ExtractMeasParam1/2(curvRate) -> IsValid2/3(curvatureRate), [curvRate]
  [curvRate] -> Subsystem1/3(curvRate)
  [curv] -> Subsystem1/2(curv)
  ExtractMeasParam1/3(curvLength) -> IsValid2/4(curvLength), [curvLen]
  ExtractMeasParam1/1(curvature) -> IsValid2/2(curvature), [curv]
  Subsystem1/1(C1) -> C1/1
  [curvLen] -> Subsystem1/4(curvLen)
  For Iterator/1 -> [index]
  ExtractMeasParam1/4(headingAngle) -> IsValid2/5(HeadingAngle), [alpha]
  ExtractMeasParam1/5(lateralOffset) -> Subsystem1/7(lateralOffset)
  Selector/1 -> For Iterator/1
  IsValid2/1(validID) -> Subsystem1/6(ValidID)
  ExtractMeasParam1/6(xmin) -> Subsystem1/8(xmin)
  CameraLineCoeff/1 -> Subsystem1/1(CameraLineCoeff)
  nLines/1 -> Selector/1
  ExtractMeasParam1/9(measCaptureTime) -> Subsystem1/11(TIME_STAMP)
  [alpha] -> Subsystem1/5(alpha)

== system FusionMODEL_version1/SENSOR_MEASUREMENTS/RADAR_CAMERA_EGO_SENSOR_INTERFACE/RoadSensors/Camera8 ==
  timeIdx : Inport
  nLines : Inport  Port=2
  CameraLineCoeff : Inport  Port=3
  ExtractMeasParam1 : Subsystem
  For Iterator : ForIterator  ResetStates=reset  IterationSource=external  IterationVariableDataType=int16
  IsValid2 : Subsystem
  Selector : Selector  InputPortWidth=nCameras  IndexOptions=Index vector (dialog)  Indices=8  OutputSizes=1
  Subsystem1 : Subsystem
  C1 : Outport
  wires:
  ExtractMeasParam1/7(xmax) -> Subsystem1/9(xmax)
  ExtractMeasParam1/8(lineMarkWidth) -> Subsystem1/10(lineWidth)
  [index] -> IsValid2/1(LineID), Subsystem1/12(iter), ExtractMeasParam1/1(idx)
  timeIdx/1 -> ExtractMeasParam1/2(time)
  ExtractMeasParam1/2(curvRate) -> IsValid2/3(curvatureRate), [curvRate]
  [curvRate] -> Subsystem1/3(curvRate)
  [curv] -> Subsystem1/2(curv)
  ExtractMeasParam1/3(curvLength) -> IsValid2/4(curvLength), [curvLen]
  ExtractMeasParam1/1(curvature) -> IsValid2/2(curvature), [curv]
  Subsystem1/1(C1) -> C1/1
  [curvLen] -> Subsystem1/4(curvLen)
  For Iterator/1 -> [index]
  ExtractMeasParam1/4(headingAngle) -> IsValid2/5(HeadingAngle), [alpha]
  ExtractMeasParam1/5(lateralOffset) -> Subsystem1/7(lateralOffset)
  Selector/1 -> For Iterator/1
  IsValid2/1(validID) -> Subsystem1/6(ValidID)
  ExtractMeasParam1/6(xmin) -> Subsystem1/8(xmin)
  CameraLineCoeff/1 -> Subsystem1/1(CameraLineCoeff)
  nLines/1 -> Selector/1
  ExtractMeasParam1/9(measCaptureTime) -> Subsystem1/11(TIME_STAMP)
  [alpha] -> Subsystem1/5(alpha)

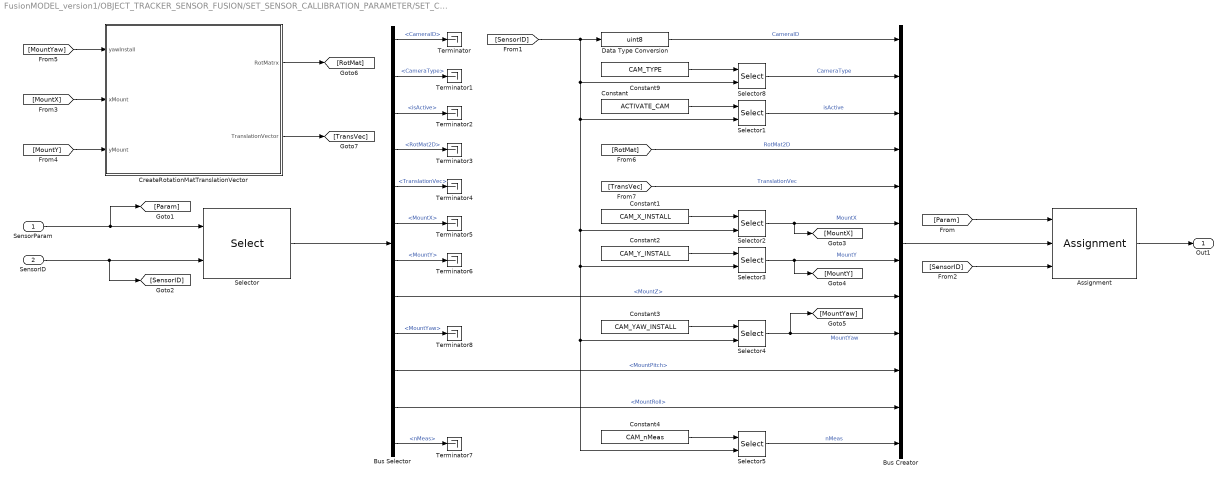
== system FusionMODEL_version1/OBJECT_TRACKER_SENSOR_FUSION/SET_SENSOR_CALLIBRATION_PARAMETER/SET_CAMERA_SENSOR_PARAM/SET_CAMERA_EXTRINSIC_PARAM/SET_CAMERA_EXTRINSIC_PARAM ==
  SensorParam : Inport
  SensorID : Inport  Port=2
  Assignment : Assignment  DiagnosticForDimensions=Warning  IndexOptions=Index vector (port)  Indices=1  OutputSizes=1
  Bus Creator : BusCreator  Inputs=12  OutDataTypeStr=Bus: CameraExtrinsicParam  NonVirtualBus=on
  Bus Selector : BusSelector  OutputSignals=CameraID,CameraType,isActive,RotMat2D,TranslationVec,MountX,MountY,MountZ,MountYaw,MountPitch,MountRoll,nMeas
  Constant : Constant  Value=ACTIVATE_CAM
  Constant1 : Constant  Value=CAM_X_INSTALL
  Constant2 : Constant  Value=CAM_Y_INSTALL
  Constant3 : Constant  Value=CAM_YAW_INSTALL
  Constant4 : Constant  Value=CAM_nMeas
  Constant9 : Constant  Value=CAM_TYPE
  CreateRotationMatTranslationVector : Subsystem
  Data Type Conversion : DataTypeConversion  OutDataTypeStr=uint8
  Selector{,1..5,8} (7 alike) : Selector  InputPortWidth=nCameras  IndexOptions=Index vector (port)  Indices=[1 3]  OutputSizes=1
  Terminator{,1..8} (9 alike) : Terminator
  Out1 : Outport
  wires:
  Assignment/1 -> Out1/1
  Constant/1 -> Selector1/1
  SensorParam/1 -> [Param], Selector/1
  Constant2/1 -> Selector3/1
  [SensorID] -> Selector5/2, Selector4/2, Selector3/2, Selector2/2, Selector1/2, Selector8/2, Data Type Conversion/1
  Constant3/1 -> Selector4/1
  Constant1/1 -> Selector2/1
  Selector/1 -> Bus Selector/1
  Bus Creator/1 -> Assignment/2
  Bus Selector/1 -> Terminator/1  "<CameraID>"
  SensorID/1 -> [SensorID], Selector/2
  [Param] -> Assignment/1
  [SensorID] -> Assignment/3
  Selector2/1 -> [MountX], Bus Creator/6  "MountX"
  Selector3/1 -> [MountY], Bus Creator/7  "MountY"
  [MountX] -> CreateRotationMatTranslationVector/2(xMount)
  [MountY] -> CreateRotationMatTranslationVector/3(yMount)
  Selector4/1 -> [MountYaw], Bus Creator/9  "MountYaw"
  [MountYaw] -> CreateRotationMatTranslationVector/1(yawInstall)
  CreateRotationMatTranslationVector/1(RotMatrx) -> [RotMat]
  CreateRotationMatTranslationVector/2(TranslationVector) -> [TransVec]
  Data Type Conversion/1 -> Bus Creator/1  "CameraID"
  Selector8/1 -> Bus Creator/2  "CameraType"
  Constant9/1 -> Selector8/1
  Selector1/1 -> Bus Creator/3  "isActive"
  [RotMat] -> Bus Creator/4  "RotMat2D"
  [TransVec] -> Bus Creator/5  "TranslationVec"
  Bus Selector/2 -> Terminator1/1  "<CameraType>"
  Bus Selector/3 -> Terminator2/1  "<isActive>"
  Bus Selector/4 -> Terminator3/1  "<RotMat2D>"
  Bus Selector/8 -> Bus Creator/8  "<MountZ>"
  Bus Selector/5 -> Terminator4/1  "<TranslationVec>"
  Bus Selector/7 -> Terminator6/1  "<MountY>"
  Bus Selector/6 -> Terminator5/1  "<MountX>"
  Bus Selector/9 -> Terminator8/1  "<MountYaw>"
  Bus Selector/11 -> Bus Creator/11  "<MountRoll>"
  Bus Selector/10 -> Bus Creator/10  "<MountPitch>"
  Selector5/1 -> Bus Creator/12  "nMeas"
  Constant4/1 -> Selector5/1
  Bus Selector/12 -> Terminator7/1  "<nMeas>"

== system FusionMODEL_version1/OBJECT_TRACKER_SENSOR_FUSION/SET_SENSOR_CALLIBRATION_PARAMETER/SET_CAMERA_SENSOR_PARAM/SET_CAMERA_INTRINSIC_PARAM/SET_CAMERA_INTRINSIC_PARAM ==
  SensorParam : Inport
  SensorID : Inport  Port=2
  Assignment : Assignment  DiagnosticForDimensions=Warning  IndexOptions=Index vector (port)  Indices=1  OutputSizes=1
  Bus Creator : BusCreator  Inputs=12  OutDataTypeStr=Bus: CameraIntrinsicParam  NonVirtualBus=on
  Bus Selector : BusSelector  OutputSignals=CameraType,RectificationMatrix,ProjectionMatrix,MaxRange,MaxAzimuth,MaxElevation,LongitudinalErrVariance,LateralErrVariance,ProbOfDetection,FalseAlarmRate,FOVRangePoints,FOVAzimuthPts
  Constant1 : Constant  Value=CAMERA_LONG_ERR_VAR
  Constant15 : Constant  Value=RADAR_PD
  Constant16 : Constant  Value=RADAR_FA
  Constant2 : Constant  Value=CAMERA_MAX_ELEVATION
  Constant3 : Constant  Value=CAMERA_LAT_ERR_VAR
  Constant4 : Constant  Value=CAMERA_MAX_RANGE
  Constant5 : Constant  Value=CAMERA_MAX_AZIMUTH
  Data Type Conversion : DataTypeConversion  OutDataTypeStr=uint8
  Selector{,1..3,5..6} (6 alike) : Selector  InputPortWidth=nCameraTypes  IndexOptions=Index vector (port)  Indices=[1 3]  OutputSizes=1
  Selector14 : Selector  InputPortWidth=nRadarTypes  IndexOptions=Index vector (port)  Indices=[1 3]  OutputSizes=1
  Selector15 : Selector  InputPortWidth=nRadarTypes  IndexOptions=Index vector (port)  Indices=[1 3]  OutputSizes=1
  Terminator{,1..7} (8 alike) : Terminator
  Out1 : Outport
  wires:
  Assignment/1 -> Out1/1
  SensorParam/1 -> [Param], Selector/1
  Selector/1 -> Bus Selector/1
  Bus Creator/1 -> Assignment/2
  SensorID/1 -> Selector/2, [SnsrTypeID]
  [Param] -> Assignment/1
  [SnsrTypeID] -> Assignment/3
  Constant5/1 -> Selector6/1
  Constant4/1 -> Selector5/1
  [SnsrTypeID] -> Selector15/2, Selector14/2, Selector3/2, Selector2/2, Selector1/2, Selector6/2, Selector5/2, Data Type Conversion/1
  Constant2/1 -> Selector1/1
  Constant15/1 -> Selector14/1
  Constant16/1 -> Selector15/1
  Bus Selector/1 -> Terminator/1  "<CameraType>"
  Bus Selector/2 -> Bus Creator/2  "<RectificationMatrix>"
  Bus Selector/4 -> Terminator3/1  "<MaxRange>"
  Bus Selector/3 -> Bus Creator/3  "<ProjectionMatrix>"
  Bus Selector/6 -> Terminator5/1  "<MaxElevation>"
  Bus Selector/7 -> Terminator6/1  "<LongitudinalErrVariance>"
  Bus Selector/8 -> Terminator7/1  "<LateralErrVariance>"
  Bus Selector/5 -> Terminator4/1  "<MaxAzimuth>"
  Selector5/1 -> Bus Creator/4  "MaxRange"
  Selector6/1 -> Bus Creator/5  "MaxAzimuth"
  Selector1/1 -> Bus Creator/6  "MaxElevation"
  Selector2/1 -> Bus Creator/7  "LongitudinalErrVariance"
  Selector3/1 -> Bus Creator/8  "LateralErrVariance"
  Constant1/1 -> Selector2/1
  Constant3/1 -> Selector3/1
  Selector14/1 -> Bus Creator/9  "ProbOfDetection"
  Selector15/1 -> Bus Creator/10  "FalseAlarmRate"
  Bus Selector/11 -> Bus Creator/11  "<FOVRangePoints>"
  Bus Selector/12 -> Bus Creator/12  "<FOVAzimuthPts>"
  Bus Selector/9 -> Terminator1/1  "<ProbOfDetection>"
  Bus Selector/10 -> Terminator2/1  "<FalseAlarmRate>"
  Data Type Conversion/1 -> Bus Creator/1  "CameraType"

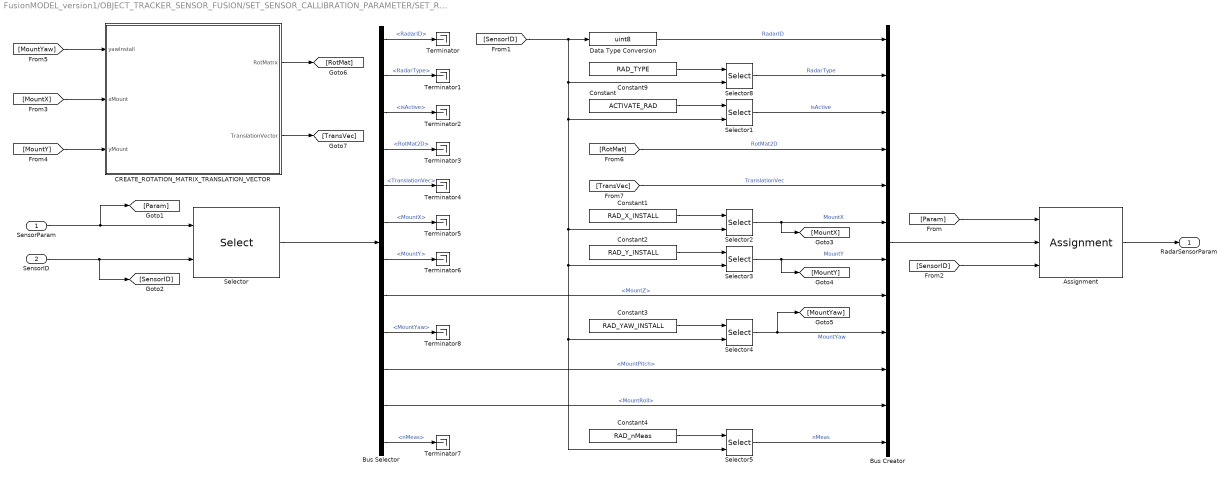
== system FusionMODEL_version1/OBJECT_TRACKER_SENSOR_FUSION/SET_SENSOR_CALLIBRATION_PARAMETER/SET_RADAR_SENSOR_PARAM/SET_RADAR_EXTRINSIC_PARAM/SET_RADAR_EXTRINSIC_PARAM ==
  SensorParam : Inport
  SensorID : Inport  Port=2
  Assignment : Assignment  DiagnosticForDimensions=Warning  IndexOptions=Index vector (port)  Indices=1  OutputSizes=1
  Bus Creator : BusCreator  Inputs=12  OutDataTypeStr=Bus: RadarExtrinsicParam  NonVirtualBus=on
  Bus Selector : BusSelector  OutputSignals=RadarID,RadarType,isActive,RotMat2D,TranslationVec,MountX,MountY,MountZ,MountYaw,MountPitch,MountRoll,nMeas
  CREATE_ROTATION_MATRIX_TRANSLATION_VECTOR : Subsystem
  Constant : Constant  Value=ACTIVATE_RAD
  Constant1 : Constant  Value=RAD_X_INSTALL
  Constant2 : Constant  Value=RAD_Y_INSTALL
  Constant3 : Constant  Value=RAD_YAW_INSTALL
  Constant4 : Constant  Value=RAD_nMeas
  Constant9 : Constant  Value=RAD_TYPE
  Data Type Conversion : DataTypeConversion  OutDataTypeStr=uint8
  Selector{,1..5,8} (7 alike) : Selector  InputPortWidth=nRadars  IndexOptions=Index vector (port)  Indices=[1 3]  OutputSizes=1
  Terminator{,1..8} (9 alike) : Terminator
  RadarSensorParam : Outport
  wires:
  Assignment/1 -> RadarSensorParam/1
  Constant/1 -> Selector1/1
  SensorParam/1 -> [Param], Selector/1
  Constant2/1 -> Selector3/1
  [SensorID] -> Selector5/2, Selector4/2, Selector3/2, Selector2/2, Selector1/2, Selector8/2, Data Type Conversion/1
  Constant3/1 -> Selector4/1
  Constant1/1 -> Selector2/1
  Selector/1 -> Bus Selector/1
  Bus Creator/1 -> Assignment/2
  Bus Selector/1 -> Terminator/1  "<RadarID>"
  SensorID/1 -> [SensorID], Selector/2
  [Param] -> Assignment/1
  [SensorID] -> Assignment/3
  Selector2/1 -> [MountX], Bus Creator/6  "MountX"
  Selector3/1 -> [MountY], Bus Creator/7  "MountY"
  [MountX] -> CREATE_ROTATION_MATRIX_TRANSLATION_VECTOR/2(xMount)
  [MountY] -> CREATE_ROTATION_MATRIX_TRANSLATION_VECTOR/3(yMount)
  Selector4/1 -> [MountYaw], Bus Creator/9  "MountYaw"
  [MountYaw] -> CREATE_ROTATION_MATRIX_TRANSLATION_VECTOR/1(yawInstall)
  CREATE_ROTATION_MATRIX_TRANSLATION_VECTOR/1(RotMatrx) -> [RotMat]
  CREATE_ROTATION_MATRIX_TRANSLATION_VECTOR/2(TranslationVector) -> [TransVec]
  Data Type Conversion/1 -> Bus Creator/1  "RadarID"
  Selector8/1 -> Bus Creator/2  "RadarType"
  Constant9/1 -> Selector8/1
  Selector1/1 -> Bus Creator/3  "isActive"
  [RotMat] -> Bus Creator/4  "RotMat2D"
  [TransVec] -> Bus Creator/5  "TranslationVec"
  Bus Selector/2 -> Terminator1/1  "<RadarType>"
  Bus Selector/3 -> Terminator2/1  "<isActive>"
  Bus Selector/4 -> Terminator3/1  "<RotMat2D>"
  Bus Selector/8 -> Bus Creator/8  "<MountZ>"
  Bus Selector/5 -> Terminator4/1  "<TranslationVec>"
  Bus Selector/7 -> Terminator6/1  "<MountY>"
  Bus Selector/6 -> Terminator5/1  "<MountX>"
  Bus Selector/9 -> Terminator8/1  "<MountYaw>"
  Bus Selector/11 -> Bus Creator/11  "<MountRoll>"
  Bus Selector/10 -> Bus Creator/10  "<MountPitch>"
  Selector5/1 -> Bus Creator/12  "nMeas"
  Constant4/1 -> Selector5/1
  Bus Selector/12 -> Terminator7/1  "<nMeas>"
